simulink model "re_servo"  (R2020b)
settings: Solver=VariableStepAuto  StartTime=0.0  StopTime=10.0  RelTol=1e-3
libraries: arduino_io_lib x4
settings Model: Creator=kei55  LastModifiedBy=kei55

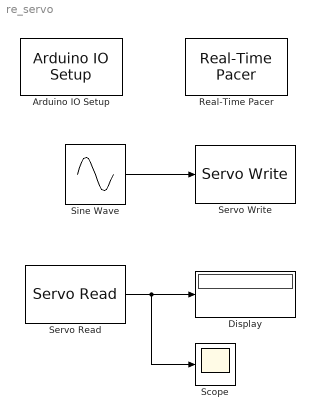
== system re_servo ==
  Arduino IO Setup : arduino_io_lib/Arduino IO Setup  Priority=3  arduinoVar=Temporary arduino variable: Arduino1  workspaceVarName=a  comPort=COM3
  Display : Display
  Real-Time Pacer : arduino_io_lib/Real-Time Pacer  simTimePerRealTime=1
  Scope : Scope
  Servo Read : arduino_io_lib/Servo Read  arduinoVar=Temporary arduino variable: Arduino1  pinNum=10  T=1/50
  Servo Write : arduino_io_lib/Servo Write  arduinoVar=Temporary arduino variable: Arduino1  pinNum=10  T=1/50
  Sine Wave : Sin  SineType=Sample based  Amplitude=45  Bias=90  Samples=100  SampleTime=1/50
  wires:
  Sine Wave/1 -> Servo Write/1
  Servo Read/1 -> Scope/1, Display/1
